simulink model "SimulinkSistemaMRA"  (R2014a)
settings: Solver=ode45  StartTime=0.0  StopTime=50  RelTol=1e-3
values from neighbouring files (symbols this model uses):
  den1 = [(j1*j2) (b2*j1+b1*j2) (k1+j2*k2+b1*b2+k2) (b1*k1+b1*k2+b2*k2) (k1*k2)]    [Coeficientes.m]
  den2 = [((j1*j2)/k2) ((1/k2)*(j2*b1+b2*j1)) (j2+((b1*b2)/k2)) (((j1*k1)/k2)+j1) (b2+((b1*k1)/k2)+b1) (1+k1-k2)]    [Coeficientes.m]
  num1 = [j2+b2 (k1+k2)]    [Coeficientes.m]
  num2 = [1]    [Coeficientes.m]
settings Model: Creator=Sala8  LastModifiedBy=Asus
settings DebuggingCC: UnderspecifiedInitializationDetection=Classic  StateNameClashWarn=warning

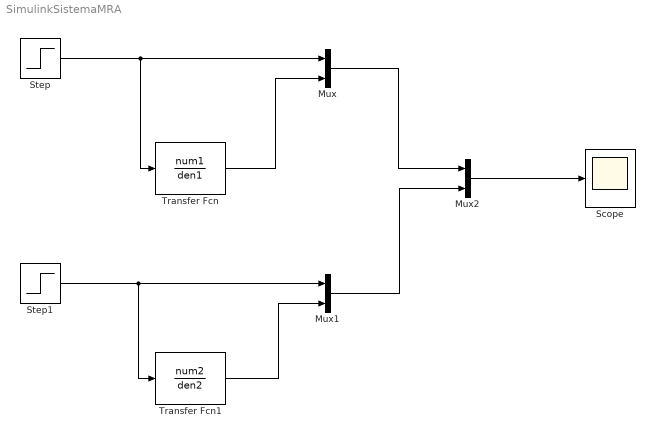
== system SimulinkSistemaMRA ==
  Mux : Mux  Inputs=2
  Mux1 : Mux  Inputs=2
  Mux2 : Mux  Inputs=2
  Scope : Scope
  Step : Step  SampleTime=0.01
  Step1 : Step  SampleTime=0.01
  Transfer Fcn : TransferFcn  Numerator=num1  Denominator=den1
  Transfer Fcn1 : TransferFcn  Numerator=num2  Denominator=den2
  wires:
  Step/1 -> Transfer Fcn/1, Mux/1
  Transfer Fcn/1 -> Mux/2
  Step1/1 -> Mux1/1, Transfer Fcn1/1
  Transfer Fcn1/1 -> Mux1/2
  Mux1/1 -> Mux2/2
  Mux/1 -> Mux2/1
  Mux2/1 -> Scope/1
